simulink model "dynamics"  (R2021b)
settings: Solver=FixedStepDiscrete  StartTime=0.0  StopTime=inf  FixedStep=0.001  RelTol=1e-3
undefined symbols (not defined in the file): DiscIntNeverNeededParam
settings Model: Creator=lywan  LastModifiedBy=lywan
settings DataIOCC: SaveFormat=Structure  SaveOutput=off
settings OptimizationCC: ZeroExternalMemoryAtStartup=off  ZeroInternalMemoryAtStartup=off
settings RTWCC: GenCodeOnly=on  Toolchain=AUTOSAR Adaptive | CMake  TargetLang=C++
settings GRTTargetCC: TargetLangStandard=C++11 (ISO)  CodeInterfacePackaging=C++ class  MultiInstanceErrorCode=None

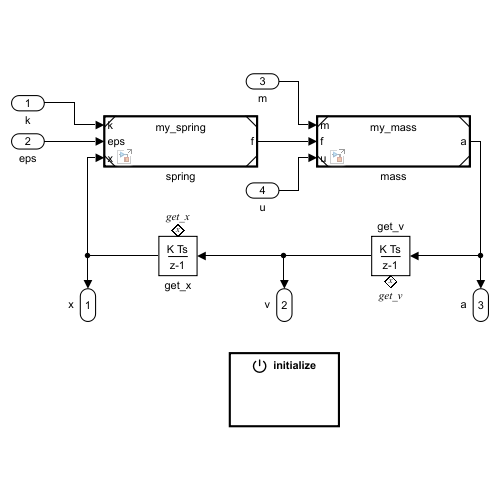
[thumbnail: Simulink's stored preview of the top-level diagram]
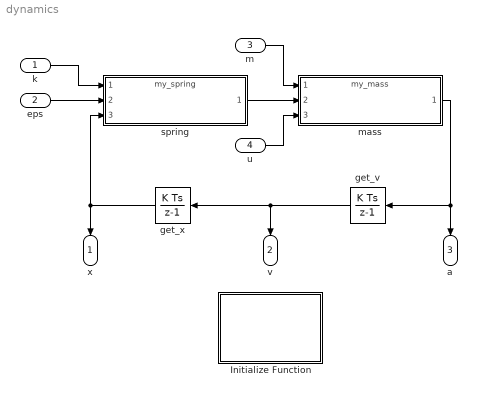
== system dynamics ==
  k : Inport
  eps : Inport  Port=2
  m : Inport  Port=3
  u : Inport  Port=4
  Initialize Function : Subsystem  TreatAsAtomicUnit=on
  get_v : DiscreteIntegrator  SampleTime=-1  ICPrevOutput=DiscIntNeverNeededParam  ICPrevScaledInput=DiscIntNeverNeededParam
  get_x : DiscreteIntegrator  SampleTime=-1  ICPrevOutput=DiscIntNeverNeededParam  ICPrevScaledInput=DiscIntNeverNeededParam
  mass : ModelReference  ModelNameDialog=my_mass.slx  SimulationMode=Normal  ModelReferenceVersion=1.6
  spring : ModelReference  ModelNameDialog=my_spring.slx  SimulationMode=Normal  ModelReferenceVersion=1.8
  x : Outport
  v : Outport  Port=2
  a : Outport  Port=3
  wires:
  spring/1 -> mass/2
  eps/1 -> spring/2
  k/1 -> spring/1
  m/1 -> mass/1
  u/1 -> mass/3
  get_v/1 -> get_x/1, v/1
  get_x/1 -> spring/3, x/1
  mass/1 -> a/1, get_v/1

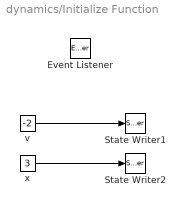
== system dynamics/Initialize Function ==
  Event Listener : EventListener  DisableCoverage=on  EventName=reset
  State Writer1 : StateWriter  StateOwnerBlock=../../get_v
  State Writer2 : StateWriter  StateOwnerBlock=../../get_x
  v : Constant  Value=-2
  x : Constant  Value=3
  wires:
  v/1 -> State Writer1/1
  x/1 -> State Writer2/1
